simulink model "rocket_landing_3d"  (R2022a)
settings: Solver=FixedStepAuto  StartTime=0.0  StopTime=10  FixedStep=0.0001  RelTol=1e-3
InitFcn:
  | model_3d_init
values from neighbouring files (symbols this model uses):
  l = 1    [model_3d_init.m]    (also in model_init.m)
  m = 1    [model_3d_init.m]    (also in model_init.m)
  phi_dot_init = 0    [model_3d_init.m]
  phi_init = 20    [model_3d_init.m]
  theta_dot_init = -10    [model_3d_init.m]    (also in model_init.m = -20)
  theta_init = 5    [model_3d_init.m]    (also in model_init.m = 20)
undefined symbols (not defined in the file or in its folder): K, magnitude, X, Y, Z
libraries: nesl_utility x15, sm_lib x7, simulink_extras x2
settings Model: Creator=Samvrit  LastModifiedBy=Samvrit
settings ExplorerConfigSet: InternalSimMechanicsExplorerSettings="<ExplorerConfiguration><canonicalview>default</canonicalview><AnimationSetting><BasePlaybackSpeed>1.0</BasePlaybackSpeed><PlaybackSpeedFactor>1.0</PlaybackSpeedFactor></AnimationSetting><TilePanel><TileInfo><Tiles Columns=\"1\" Count=\"1\" Rows=\"1\"><Column Weight=\"1\"/><Row Weight=\"1\"/><Tile Height=\"1\" Width=\"1\" X=\"0\" Y=\"0\"/></Tiles></TileInfo><SceneInfo><SceneViewer><BGColor><R>0.60000002384185791</R><G>0.60000002384185791</G><B>0.60000002384185791</B></BGColor><Camera><DoPerspective>off</DoPerspective><Position><X>0.449860961652100377</X><Y>1.73634806116314278</Y><Z>2.29390141757635169</Z></Position><Center><X>0.371440472231759244</X><Y>1.38468287874813889</Y><Z>-0.111192153708824293</Z></Center><Up><X>-0.00855771250830794118</X><Y>0.989482399018140057</Y><Z>-0.144399957028844561</Z></Up><ViewLimDist>1</ViewLimDist><YLim>1.53478052056081382</YLim><XLim>1.66025162881104094</XLim></Camera></SceneViewer></SceneInfo></TilePanel><MechEditorPanel><Cameras/><GfxPanelCameraMap/><VideoCreator><PlaybackSpeedRatio>1.0</PlaybackSpeedRatio><FrameRate>30</FrameRate><VideoFormat>MPEG-4</VideoFormat><FrameSize>[1920 1080]</FrameSize></VideoCreator></MechEditorPanel></ExplorerConfiguration>"

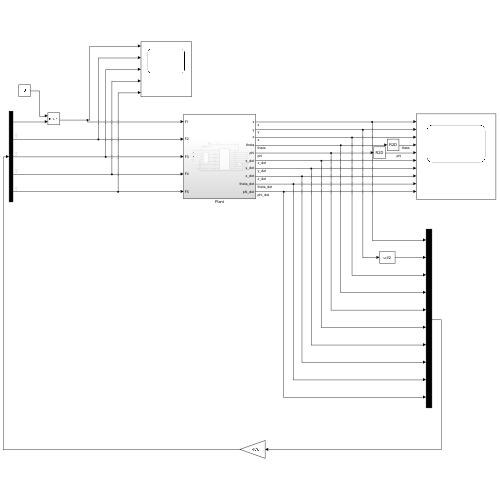
[thumbnail: Simulink's stored preview of the top-level diagram]
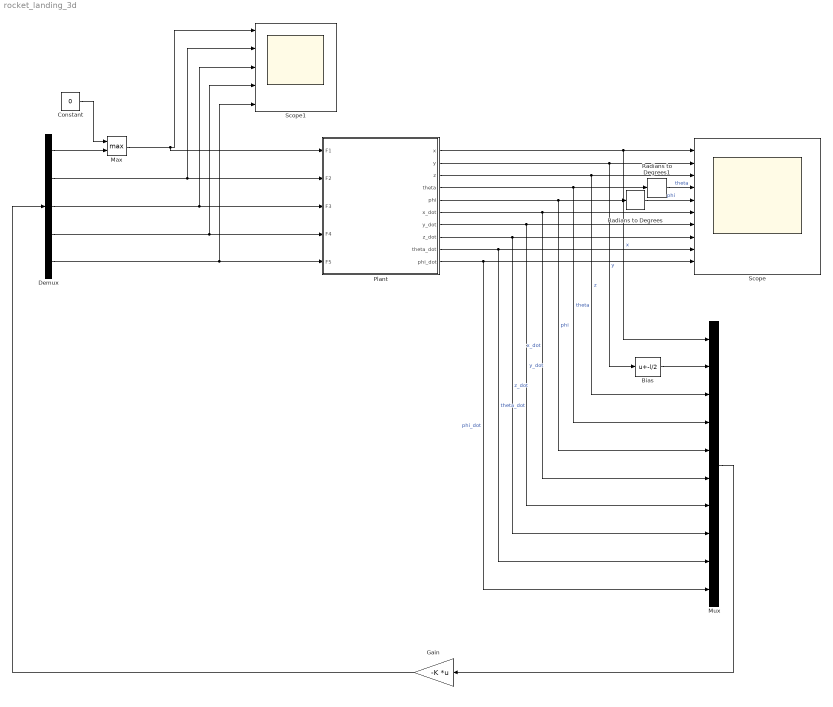
== system rocket_landing_3d ==
  Bias : Bias  Bias=-l/2  SaturateOnIntegerOverflow=off
  Constant : Constant  Value=0
  Demux : Demux  Outputs=5
  Gain : Gain  Gain=-K  Multiplication=Matrix(K*u)
  Max : MinMax  Function=max  Inputs=2
  Mux : Mux  Inputs=10
  Plant : Subsystem
  Radians to Degrees : simulink_extras/Transformations/Radians to Degrees
  Radians to Degrees1 : simulink_extras/Transformations/Radians to Degrees
  Scope : Scope  NumInputPorts=10
  Scope1 : Scope  NumInputPorts=5
  wires:
  Mux/1 -> Gain/1
  Bias/1 -> Mux/2
  Plant/1(x) -> Mux/1, Scope/1  "x"
  Plant/2(y) -> Bias/1, Scope/2  "y"
  Plant/3(z) -> Mux/3, Scope/3  "z"
  Plant/4(theta) -> Mux/4, Radians to Degrees1/1  "theta"
  Plant/5(phi) -> Mux/5, Radians to Degrees/1  "phi"
  Plant/6(x_dot) -> Mux/6, Scope/6  "x_dot"
  Plant/7(y_dot) -> Mux/7, Scope/7  "y_dot"
  Plant/8(z_dot) -> Mux/8, Scope/8  "z_dot"
  Plant/9(theta_dot) -> Mux/9, Scope/9  "theta_dot"
  Plant/10(phi_dot) -> Mux/10, Scope/10  "phi_dot"
  Demux/1 -> Max/2
  Constant/1 -> Max/1
  Max/1 -> Plant/1(F1), Scope1/1
  Demux/2 -> Plant/2(F2), Scope1/2
  Demux/3 -> Scope1/3, Plant/3(F3)
  Demux/5 -> Plant/5(F5), Scope1/5
  Demux/4 -> Plant/4(F4), Scope1/4
  Radians to Degrees1/1 -> Scope/4  "theta"
  Radians to Degrees/1 -> Scope/5  "phi"
  Gain/1 -> Demux/1

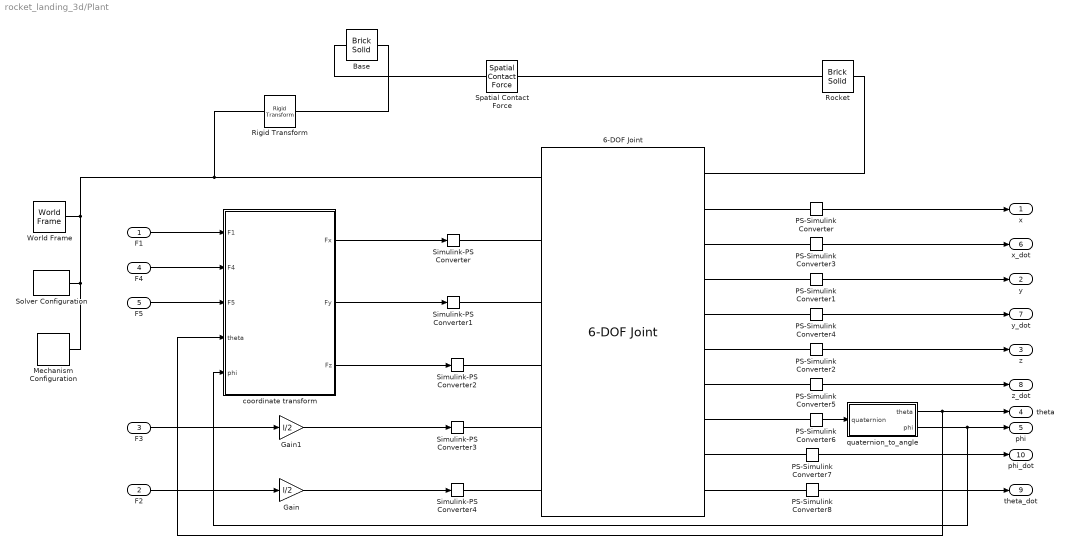
== system rocket_landing_3d/Plant ==
  F1 : Inport
  F2 : Inport  Port=2
  F3 : Inport  Port=3
  F4 : Inport  Port=4
  F5 : Inport  Port=5
  6-DOF Joint : sm_lib/Joints/6-DOF Joint  JointMode=Normal  SenseConstraintForce=off  SenseConstraintForceX=off  SenseConstraintForceY=off  SenseConstraintForceZ=off  SenseConstraintTorque=off  SenseConstraintTorqueX=off  SenseConstraintTorqueY=off  SenseConstraintTorqueZ=off  SenseTotalForce=off  SenseTotalForceX=off  SenseTotalForceY=off  SenseTotalForceZ=off  SenseTotalTorque=off  SenseTotalTorqueX=off  SenseTotalTorqueY=off  SenseTotalTorqueZ=off  CompositeWrenchDir=FollowerOnBase  CompositeWrenchFrame=BaseFrame  PxEquilibriumPosition=0  PxEquilibriumPositionUnits=m  PxSpringStiffness=0  PxSpringStiffnessUnits=N/m  PxDampingCoefficient=0  PxDampingCoefficientUnits=N/(m/s)  PxTorqueActuationMode=InputTorque  PxMotionActuationMode=ComputedMotion  PxSensePosition=on  PxSenseVelocity=on  PxSenseAcceleration=off  PxSenseTorqueForce=off  PxSenseLowerLimitTorqueForce=off  PxSenseUpperLimitTorqueForce=off  PxLowerLimitSpecify=off  PxLowerLimitBound=-1  PxLowerLimitBoundUnits=m  PxLowerLimitStiffness=1e6  PxLowerLimitStiffnessUnits=N/m  PxLowerLimitDamping=1e3  PxLowerLimitDampingUnits=N/(m/s)  PxLowerLimitTransitionRegionWidth=1e-4  PxLowerLimitTransitionRegionWidthUnits=m  PxUpperLimitSpecify=off  PxUpperLimitBound=1  PxUpperLimitBoundUnits=m  PxUpperLimitStiffness=1e6  PxUpperLimitStiffnessUnits=N/m  PxUpperLimitDamping=1e3  PxUpperLimitDampingUnits=N/(m/s)  PxUpperLimitTransitionRegionWidth=1e-4  PxUpperLimitTransitionRegionWidthUnits=m  PxPositionTargetSpecify=on  PxPositionTargetPriority=High  PxPositionTargetValue=x_init  PxPositionTargetValueUnits=m  PxVelocityTargetSpecify=on  PxVelocityTargetPriority=High  PxVelocityTargetValue=x_dot_init  PxVelocityTargetValueUnits=m/s  PyEquilibriumPosition=0  PyEquilibriumPositionUnits=m  PySpringStiffness=0  PySpringStiffnessUnits=N/m  PyDampingCoefficient=0  PyDampingCoefficientUnits=N/(m/s)  PyTorqueActuationMode=InputTorque  PyMotionActuationMode=ComputedMotion  PySensePosition=on  PySenseVelocity=on  PySenseAcceleration=off  PySenseTorqueForce=off  PySenseLowerLimitTorqueForce=off  PySenseUpperLimitTorqueForce=off  PyLowerLimitSpecify=off  PyLowerLimitBound=-1  PyLowerLimitBoundUnits=m  PyLowerLimitStiffness=1e6  PyLowerLimitStiffnessUnits=N/m  PyLowerLimitDamping=1e3  PyLowerLimitDampingUnits=N/(m/s)  PyLowerLimitTransitionRegionWidth=1e-4  PyLowerLimitTransitionRegionWidthUnits=m  PyUpperLimitSpecify=off  PyUpperLimitBound=1  PyUpperLimitBoundUnits=m  PyUpperLimitStiffness=1e6  PyUpperLimitStiffnessUnits=N/m  PyUpperLimitDamping=1e3  PyUpperLimitDampingUnits=N/(m/s)  PyUpperLimitTransitionRegionWidth=1e-4  PyUpperLimitTransitionRegionWidthUnits=m  PyPositionTargetSpecify=on  PyPositionTargetPriority=High  PyPositionTargetValue=y_init  PyPositionTargetValueUnits=m  PyVelocityTargetSpecify=on  PyVelocityTargetPriority=High  PyVelocityTargetValue=y_dot_init  PyVelocityTargetValueUnits=m/s  PzEquilibriumPosition=0  PzEquilibriumPositionUnits=m  PzSpringStiffness=0  PzSpringStiffnessUnits=N/m  PzDampingCoefficient=0  PzDampingCoefficientUnits=N/(m/s)  PzTorqueActuationMode=InputTorque  PzMotionActuationMode=ComputedMotion  PzSensePosition=on  PzSenseVelocity=on  PzSenseAcceleration=off  PzSenseTorqueForce=off  PzSenseLowerLimitTorqueForce=off  PzSenseUpperLimitTorqueForce=off  PzLowerLimitSpecify=off  PzLowerLimitBound=-1  PzLowerLimitBoundUnits=m  PzLowerLimitStiffness=1e6  PzLowerLimitStiffnessUnits=N/m  PzLowerLimitDamping=1e3  PzLowerLimitDampingUnits=N/(m/s)  PzLowerLimitTransitionRegionWidth=1e-4  PzLowerLimitTransitionRegionWidthUnits=m  PzUpperLimitSpecify=off  PzUpperLimitBound=1  PzUpperLimitBoundUnits=m  PzUpperLimitStiffness=1e6  PzUpperLimitStiffnessUnits=N/m  PzUpperLimitDamping=1e3  PzUpperLimitDampingUnits=N/(m/s)  PzUpperLimitTransitionRegionWidth=1e-4  PzUpperLimitTransitionRegionWidthUnits=m  PzPositionTargetSpecify=on  PzPositionTargetPriority=High  PzPositionTargetValue=z_init  PzPositionTargetValueUnits=m  PzVelocityTargetSpecify=on  PzVelocityTargetPriority=High  PzVelocityTargetValue=z_dot_init  PzVelocityTargetValueUnits=m/s  SphDefPosRotationMethod=None  SphDefPosRotationAngleUnits=deg  SphDefPosRotationStandardAxis=+Z  SphDefPosRotationAngle=0.0  SphDefPosRotationArbitraryAxis=[0 0 1]  SphDefPosFollAlignAxisA=+X  SphDefPosBaseAlignAxisA=+Y  SphDefPosFollAlignAxisB=+Y  SphDefPosBaseAlignAxisB=+Z  SphDefPosRotationSequenceAxes=FollowerAxes  SphDefPosRotationSequence=XYX  SphDefPosRotationSequenceAngles=[0 0 0]  SphDefPosRotationSequenceAnglesUnits=deg  SphDefPosRotationMatrix=[1 0 0; 0 1 0; 0 0 1]  SphEqPosRotationMethod=None  SphEqPosRotationAngleUnits=deg  SphEqPosRotationStandardAxis=+Z  SphEqPosRotationAngle=0.0  SphEqPosRotationArbitraryAxis=[0 0 1]  SphEqPosFollAlignAxisA=+X  SphEqPosBaseAlignAxisA=+Y  SphEqPosFollAlignAxisB=+Y  SphEqPosBaseAlignAxisB=+Z  SphEqPosRotationSequenceAxes=FollowerAxes  SphEqPosRotationSequence=XYX  SphEqPosRotationSequenceAngles=[0 0 0]  SphEqPosRotationSequenceAnglesUnits=deg  SphEqPosRotationMatrix=[1 0 0; 0 1 0; 0 0 1]  SphSpringStiffness=0  SphSpringStiffnessUnits=N*m/deg  SphDampingCoefficient=0  SphDampingCoefficientUnits=N*m/(deg/s)  SphActuateTorqueX=on  SphActuateTorqueY=off  SphActuateTorqueZ=on  SphActuateTorque=off  SphTorqueActuationMode=InputTorque  SphMotionActuationMode=ComputedMotion  SphActuationFrame=FollowerFrame  SphSensePosition=on  SphSenseVelocityX=on  SphSenseVelocityY=off  SphSenseVelocityZ=on  SphSenseVelocity=off  SphSenseAccelerationX=off  SphSenseAccelerationY=off  SphSenseAccelerationZ=off  SphSenseAcceleration=off  SphSenseTorqueX=off  SphSenseTorqueY=off  SphSenseTorqueZ=off  SphSenseTorqueForce=off  SphSenseLowerLimitTorqueMag=off  SphSenseUpperLimitTorqueMag=off  SphSensingFrame=FollowerFrame  SphLowerLimitSpecify=off  SphLowerLimitBound=15  SphLowerLimitBoundUnits=deg  SphLowerLimitStiffness=1e4  SphLowerLimitStiffnessUnits=N*m/deg  SphLowerLimitDamping=10  SphLowerLimitDampingUnits=N*m/(deg/s)  SphLowerLimitTransitionRegionWidth=0.1  SphLowerLimitTransitionRegionWidthUnits=deg  SphUpperLimitSpecify=off  SphUpperLimitBound=45  SphUpperLimitBoundUnits=deg  SphUpperLimitStiffness=1e4  SphUpperLimitStiffnessUnits=N*m/deg  SphUpperLimitDamping=10  SphUpperLimitDampingUnits=N*m/(deg/s)  SphUpperLimitTransitionRegionWidth=0.1  SphUpperLimitTransitionRegionWidthUnits=deg  SphPositionTargetRotationMethod=RotationSequence  SphPositionTargetRotationAngleUnits=deg  SphPositionTargetRotationStandardAxis=+Z  SphPositionTargetRotationAngle=theta_init  SphPositionTargetRotationArbitraryAxis=[0 0 1]  SphPositionTargetFollAlignAxisA=+X  SphPositionTargetBaseAlignAxisA=+Y  SphPositionTargetFollAlignAxisB=+Y  SphPositionTargetBaseAlignAxisB=+Z  SphPositionTargetRotationSequenceAxes=FollowerAxes  SphPositionTargetRotationSequence=ZXY  SphPositionTargetRotationSequenceAngles=[theta_init phi_init 0]  SphPositionTargetRotationSequenceAnglesUnits=deg  SphPositionTargetRotationMatrix=[1 0 0; 0 1 0; 0 0 1]  SphPositionTargetSpecify=on  SphPositionTargetPriority=High  SphVelocityTargetValue=[phi_dot_init 0 theta_dot_init]  SphVelocityTargetValueUnits=deg/s  SphVelocityTargetSpecify=on  SphVelocityTargetPriority=High  SphVelocityTargetInFollowerFrame=on
  Base : sm_lib/Body Elements/Brick Solid  GraphicAmbientColor=[0.15 0.15 0.15 1.0]  BasedOnType=Density  BrickDimensions=[1 0.05 1]  BrickDimensionUnits=m  CenterOfMass=[0 0 0]  CenterOfMassUnits=m  GraphicDiffuseColor=[0.2 0.0 0.0]  Density=1000  DensityUnits=kg/m^3  DoExposeReferenceFrame=on  GraphicEmissiveColor=[0.0 0.0 0.0 1.0]  ExportEntireGeometry=on  SerializedFrames=<Frames/>  MarkerShape=Sphere  MarkerSize=10  GraphicType=FromGeometry  InertiaType=CalculateFromGeometry  Mass=1  MassUnits=kg  MomentsOfInertia=[1 1 1]  MomentsOfInertiaUnits=kg*m^2  GraphicOpacity=1.0  ProductsOfInertia=[0 0 0]  ProductsOfInertiaUnits=kg*m^2  GraphicShininess=75  GraphicSpecularColor=[0.5 0.5 0.5 1.0]  GraphicVisPropType=SimpleVisualProperties
  Gain : Gain  Gain=l/2
  Gain1 : Gain  Gain=l/2
  Mechanism Configuration : sm_lib/Utilities/Mechanism Configuration  UniformGravity=Constant  GravityVector=[0 -9.81 0]  GravityUnits=m/s^2  LinearizationDelta=0.001  JointModeTransitionNonlinearIterations=2
  PS-Simulink Converter{,1..8} (9 alike) : nesl_utility/PS-Simulink Converter  PhysicalDomain=network_engine_domain  SubClassName=ps_output  LeftPortType=input  RightPortType=output  PseudoPeriodic=off  Frequencies=[]  VectorFormat=inherit  Unit=inherit  AffineConversion=off
      settings: SourceProductBaseCode=SS,PW,VE
  Rigid Transform : sm_lib/Frames and Transforms/Rigid Transform  TranslationMethod=StandardAxis  TranslationStandardOffset=0.025  TranslationLengthUnit=m  TranslationStandardAxis=-Y  TranslationCartesianOffset=[0 0 0]  TranslationROffset=0  TranslationROffsetUnits=m  TranslationZOffset=0  TranslationZOffsetUnits=m  TranslationThetaOffset=0  TranslationThetaOffsetUnits=deg  RotationMethod=None  RotationAngleUnits=deg  RotationStandardAxis=+Z  RotationAngle=0.0  RotationArbitraryAxis=[0 0 1]  FollAlignAxisA=+X  BaseAlignAxisA=+Y  FollAlignAxisB=+Y  BaseAlignAxisB=+Z  RotationSequenceAxes=FollowerAxes  RotationSequence=XYX  RotationSequenceAngles=[0 0 0]  RotationSequenceAnglesUnits=deg  RotationMatrix=[1 0 0; 0 1 0; 0 0 1]
  Rocket : sm_lib/Body Elements/Brick Solid  GraphicAmbientColor=[0.15 0.15 0.15 1.0]  BasedOnType=Density  BrickDimensions=[sqrt(0.001) l sqrt(0.001)]  BrickDimensionUnits=m  CenterOfMass=[0 0 0]  CenterOfMassUnits=m  GraphicDiffuseColor=[1.0 0.0 0.2]  Density=1000  DensityUnits=kg/m^3  DoExposeReferenceFrame=on  GraphicEmissiveColor=[0.0 0.0 0.0 1.0]  ExportEntireGeometry=on  SerializedFrames=<Frames/>  MarkerShape=Sphere  MarkerSize=10  GraphicType=FromGeometry  InertiaType=CalculateFromGeometry  Mass=1  MassUnits=kg  MomentsOfInertia=[1 1 1]  MomentsOfInertiaUnits=kg*m^2  GraphicOpacity=1.0  ProductsOfInertia=[0 0 0]  ProductsOfInertiaUnits=kg*m^2  GraphicShininess=75  GraphicSpecularColor=[0.5 0.5 0.5 1.0]  GraphicVisPropType=SimpleVisualProperties
  Simulink-PS Converter{,1..4} (5 alike) : nesl_utility/Simulink-PS Converter  PhysicalDomain=network_engine_domain  SubClassName=ps_input  LeftPortType=input  RightPortType=output  PseudoPeriodic=off  Frequencies=[]  NoiseDistribution=none  NoiseParameters=[]  Unit=1  AffineConversion=off  FilteringAndDerivatives=provide  SimscapeFilterOrder=1  InputFilterTimeConstant=0.001  UdotUserProvided=0
      settings: SourceProductBaseCode=SS,PW,VE
  Solver Configuration : nesl_utility/Solver Configuration  PhysicalDomain=network_engine_domain  SubClassName=solver  LeftPortType=input  RightPortType=generic  Tones=[]  Harmonics=[]  SimulateNoise=off  Profile=off  UseLocalSampling=off  EnableSwitchedLinearOptims=on  FrequencyDomain=off  UseCCode=off  RelTol=0.001  AbsTol=0.001  MinStep=1e-09  ToWorkspace=off  RevertToSquareIcSolve=off  NumHomotopyIterations=100  PhasorMode=off  PhasorModeNumHarmonics=1  IndexReductionMethod=DerivativeReplacement  DoDC=off  ResidualTolerance=1e-09  UseLocalSolver=on  LocalSolverChoice=NE_BACKWARD_EULER_ADVANCER  LocalSolverSampleTime=0.0001  DoFixedCost=on  MaxNonlinIter=3  MaxModeIter=2  ComputeImpulses=off  ImpulseIterations=2  LinearAlgebra=auto  LinearAlgebraNumThread=0  EquationFormulation=NE_TIME_EF  DelaysMemoryBudget=1024  AutomaticFiltering=on  FilteringTimeConstant=0.001  PartitionStorageMethod=AS_NEEDED  PartitionMemoryBudget=1024  PartitionMethod=ROBUST
      settings: SourceProductBaseCode=SS,PW,VE
  Spatial Contact Force : sm_lib/Forces and Torques/Spatial Contact Force  SenseContactBaseRotation=off  SenseContactBaseTranslation=off  CoefficientOfDynamicFriction=0.3  CoefficientOfStaticFriction=0.5  NormalDamping=1e3  NormalDampingUnits=N/(m/s)  SenseContactSignal=off  NormalStiffness=1e6  NormalStiffnessUnits=N/m  FrictionalCriticalVelocity=1e-3  FrictionalCriticalVelocityUnits=m/s  ZeroCrossDetectContactStartAndEnd=off  SenseContactFollowerRotation=off  SenseContactFollowerTranslation=off  FrictionType=SmoothStickSlip  SenseFrictionalForceMagnitude=off  SenseNormalForceMagnitude=off  NormalForceType=SmoothSpringDamper  SenseNormalVelocity=off  SenseSeparationDistance=off  SenseTangentialVelocity=off  NormalTransitionRegionWidth=1e-4  NormalTransitionRegionWidthUnits=m
  World Frame : sm_lib/Frames and Transforms/World Frame
  coordinate transform : Subsystem
  quaternion_to_angle : Subsystem
  x : Outport
  y : Outport  Port=2
  z : Outport  Port=3
  theta : Outport  Port=4
  phi : Outport  Port=5
  x_dot : Outport  Port=6
  y_dot : Outport  Port=7
  z_dot : Outport  Port=8
  theta_dot : Outport  Port=9
  phi_dot : Outport  Port=10
  wires:
  PS-Simulink Converter5/1 -> z_dot/1
  PS-Simulink Converter3/1 -> x_dot/1
  PS-Simulink Converter4/1 -> y_dot/1
  PS-Simulink Converter/1 -> x/1
  PS-Simulink Converter1/1 -> y/1
  PS-Simulink Converter2/1 -> z/1
  PS-Simulink Converter6/1 -> quaternion_to_angle/1(quaternion)
  quaternion_to_angle/2(phi) -> coordinate transform/5(phi), phi/1
  PS-Simulink Converter8/1 -> theta_dot/1
  PS-Simulink Converter7/1 -> phi_dot/1
  coordinate transform/1(Fx) -> Simulink-PS Converter/1
  coordinate transform/2(Fy) -> Simulink-PS Converter1/1
  coordinate transform/3(Fz) -> Simulink-PS Converter2/1
  Gain1/1 -> Simulink-PS Converter3/1
  Gain/1 -> Simulink-PS Converter4/1
  quaternion_to_angle/1(theta) -> coordinate transform/4(theta), theta/1
  F2/1 -> Gain/1
  F3/1 -> Gain1/1
  F1/1 -> coordinate transform/1(F1)
  F4/1 -> coordinate transform/2(F4)
  F5/1 -> coordinate transform/3(F5)
  connections:
  World Frame/RConn1 -- Rigid Transform/LConn1 -- 6-DOF Joint/LConn1 -- Mechanism Configuration/RConn1 -- Solver Configuration/RConn1
  6-DOF Joint/RConn5 -- PS-Simulink Converter4/LConn1
  PS-Simulink Converter3/LConn1 -- 6-DOF Joint/RConn3
  PS-Simulink Converter1/LConn1 -- 6-DOF Joint/RConn4
  6-DOF Joint/RConn1 -- Rocket/RConn1
  Simulink-PS Converter/RConn1 -- 6-DOF Joint/LConn2
  PS-Simulink Converter/LConn1 -- 6-DOF Joint/RConn2
  6-DOF Joint/RConn6 -- PS-Simulink Converter2/LConn1
  Simulink-PS Converter1/RConn1 -- 6-DOF Joint/LConn3
  PS-Simulink Converter5/LConn1 -- 6-DOF Joint/RConn7
  Simulink-PS Converter2/RConn1 -- 6-DOF Joint/LConn4
  Simulink-PS Converter3/RConn1 -- 6-DOF Joint/LConn5
  PS-Simulink Converter6/LConn1 -- 6-DOF Joint/RConn8
  PS-Simulink Converter7/LConn1 -- 6-DOF Joint/RConn9
  PS-Simulink Converter8/LConn1 -- 6-DOF Joint/RConn10
  Simulink-PS Converter4/RConn1 -- 6-DOF Joint/LConn6
  Base/RConn1 -- Rigid Transform/RConn1
  Spatial Contact Force/LConn1 -- Base/LConn1
  Rocket/LConn1 -- Spatial Contact Force/RConn1

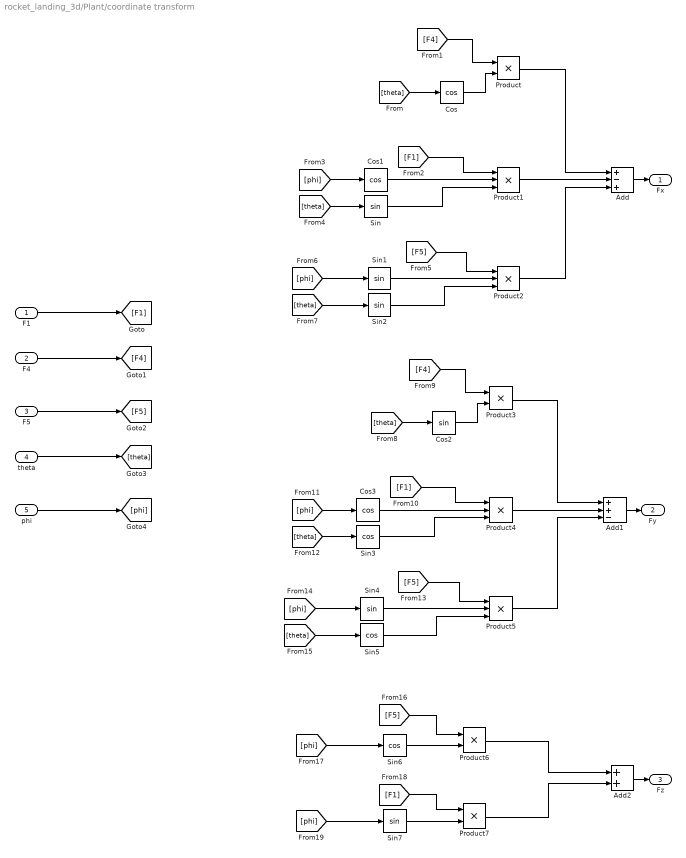
== system rocket_landing_3d/Plant/coordinate transform ==
  F1 : Inport
  F4 : Inport  Port=2
  F5 : Inport  Port=3
  theta : Inport  Port=4
  phi : Inport  Port=5
  Add : Sum  Inputs=+-+
  Add1 : Sum  Inputs=++-
  Add2 : Sum
  Cos : Trigonometry  Operator=cos
  Cos1 : Trigonometry  Operator=cos
  Cos2 : Trigonometry
  Cos3 : Trigonometry  Operator=cos
  Product{,3,6..7} (4 alike) : Product
  Product{1..2,4..5} (4 alike) : Product  Inputs=3
  Sin{,1..2,4,7} (5 alike) : Trigonometry
  Sin3 : Trigonometry  Operator=cos
  Sin5 : Trigonometry  Operator=cos
  Sin6 : Trigonometry  Operator=cos
  Fx : Outport
  Fy : Outport  Port=2
  Fz : Outport  Port=3
  wires:
  [theta] -> Cos/1
  Product7/1 -> Add2/2
  Sin7/1 -> Product7/2
  Sin/1 -> Product1/3
  [phi] -> Sin7/1
  Product6/1 -> Add2/1
  Sin2/1 -> Product2/3
  Sin4/1 -> Product5/2
  [theta] -> Sin2/1
  [phi] -> Sin6/1
  [theta] -> Sin/1
  [theta] -> Sin5/1
  [F4] -> Product/1
  [F1] -> Product1/1
  Cos2/1 -> Product3/2
  Product3/1 -> Add1/1
  Sin5/1 -> Product5/3
  Cos1/1 -> Product1/2
  [phi] -> Cos1/1
  Product2/1 -> Add/3
  [F5] -> Product2/1
  Cos/1 -> Product/2
  Product5/1 -> Add1/3
  [F5] -> Product5/1
  [F4] -> Product3/1
  [phi] -> Sin1/1
  Product/1 -> Add/1
  Sin1/1 -> Product2/2
  [phi] -> Sin4/1
  Product1/1 -> Add/2
  Product4/1 -> Add1/2
  Sin6/1 -> Product6/2
  [F1] -> Product4/1
  [F5] -> Product6/1
  [theta] -> Cos2/1
  Sin3/1 -> Product4/3
  [theta] -> Sin3/1
  Cos3/1 -> Product4/2
  [phi] -> Cos3/1
  [F1] -> Product7/1
  Add/1 -> Fx/1
  Add1/1 -> Fy/1
  Add2/1 -> Fz/1
  F5/1 -> [F5]
  F4/1 -> [F4]
  F1/1 -> [F1]
  theta/1 -> [theta]
  phi/1 -> [phi]

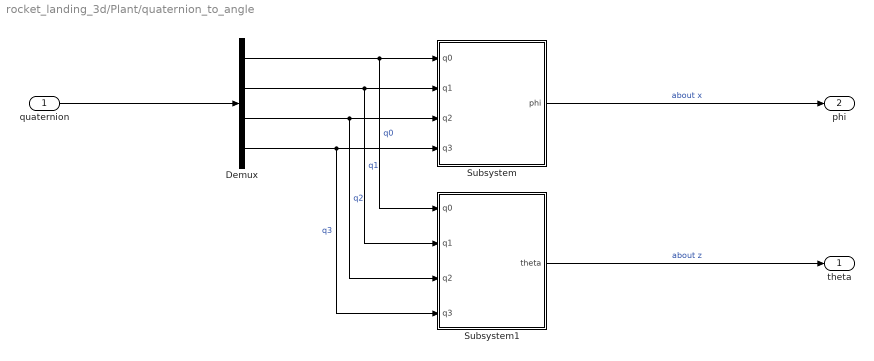
== system rocket_landing_3d/Plant/quaternion_to_angle ==
  quaternion : Inport
  Demux : Demux
  Subsystem : Subsystem
  Subsystem1 : Subsystem
  theta : Outport
  phi : Outport  Port=2
  wires:
  quaternion/1 -> Demux/1
  Demux/1 -> Subsystem1/1(q0), Subsystem/1(q0)  "q0"
  Demux/2 -> Subsystem1/2(q1), Subsystem/2(q1)  "q1"
  Demux/3 -> Subsystem1/3(q2), Subsystem/3(q2)  "q2"
  Demux/4 -> Subsystem1/4(q3), Subsystem/4(q3)  "q3"
  Subsystem1/1(theta) -> theta/1  "about z"
  Subsystem/1(phi) -> phi/1  "about x"

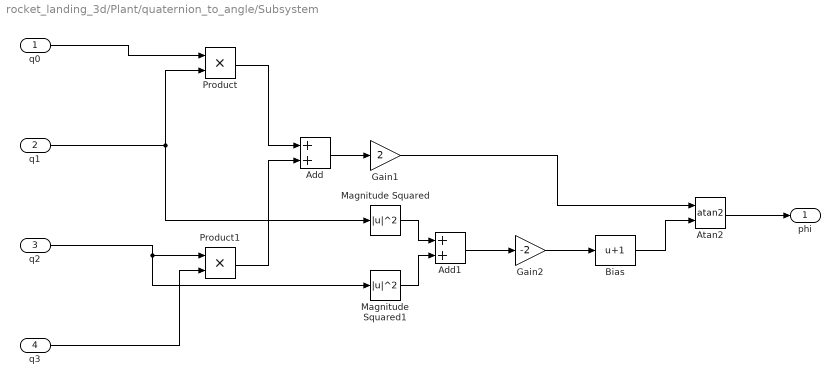
== system rocket_landing_3d/Plant/quaternion_to_angle/Subsystem ==
  q0 : Inport
  q1 : Inport  Port=2
  q2 : Inport  Port=3
  q3 : Inport  Port=4
  Add : Sum
  Add1 : Sum
  Atan2 : Trigonometry  Operator=atan2
  Bias : Bias  Bias=1  SaturateOnIntegerOverflow=off
  Gain1 : Gain  Gain=2
  Gain2 : Gain  Gain=-2
  Magnitude Squared : Math  Operator=magnitude^2
  Magnitude Squared1 : Math  Operator=magnitude^2
  Product : Product
  Product1 : Product
  phi : Outport
  wires:
  Gain2/1 -> Bias/1
  Gain1/1 -> Atan2/1
  Product1/1 -> Add/2
  Add1/1 -> Gain2/1
  Product/1 -> Add/1
  q1/1 -> Product/2, Magnitude Squared/1
  Magnitude Squared1/1 -> Add1/2
  Add/1 -> Gain1/1
  Magnitude Squared/1 -> Add1/1
  Atan2/1 -> phi/1
  q2/1 -> Magnitude Squared1/1, Product1/1
  Bias/1 -> Atan2/2
  q0/1 -> Product/1
  q3/1 -> Product1/2

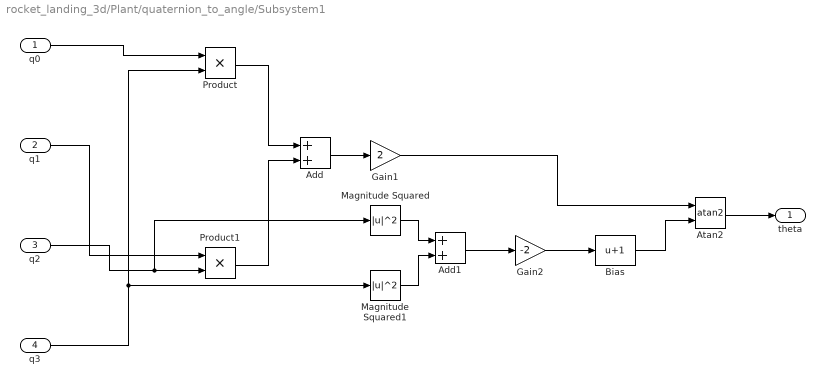
== system rocket_landing_3d/Plant/quaternion_to_angle/Subsystem1 ==
  q0 : Inport
  q1 : Inport  Port=2
  q2 : Inport  Port=3
  q3 : Inport  Port=4
  Add : Sum
  Add1 : Sum
  Atan2 : Trigonometry  Operator=atan2
  Bias : Bias  Bias=1  SaturateOnIntegerOverflow=off
  Gain1 : Gain  Gain=2
  Gain2 : Gain  Gain=-2
  Magnitude Squared : Math  Operator=magnitude^2
  Magnitude Squared1 : Math  Operator=magnitude^2
  Product : Product
  Product1 : Product
  theta : Outport
  wires:
  Bias/1 -> Atan2/2
  Atan2/1 -> theta/1
  Magnitude Squared/1 -> Add1/1
  Add/1 -> Gain1/1
  Magnitude Squared1/1 -> Add1/2
  Product/1 -> Add/1
  Add1/1 -> Gain2/1
  Product1/1 -> Add/2
  Gain1/1 -> Atan2/1
  Gain2/1 -> Bias/1
  q0/1 -> Product/1
  q3/1 -> Magnitude Squared1/1, Product/2
  q1/1 -> Product1/1
  q2/1 -> Magnitude Squared/1, Product1/2
